simulink model "ident"  (R2018a)
settings: Solver=FixedStepAuto  StartTime=0.0  StopTime=1000  FixedStep=1e-2  MaxStep=1e-2  RelTol=1e-3
values from neighbouring files (symbols this model uses):
  B = 1    [data.m]
  C = 5    [data.m]
  V1 = 10    [data.m]
  V2 = 20    [data.m]
settings Model: Creator=User  LastModifiedBy=User

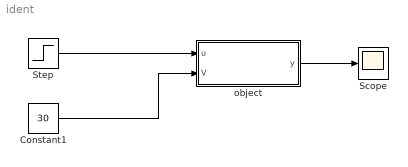
== system ident ==
  Constant1 : Constant  Value=30
  Scope : Scope
  Step : Step  SampleTime=0.01
  object : Subsystem
  wires:
  Constant1/1 -> object/2(V)
  Step/1 -> object/1(u)
  object/1(y) -> Scope/1

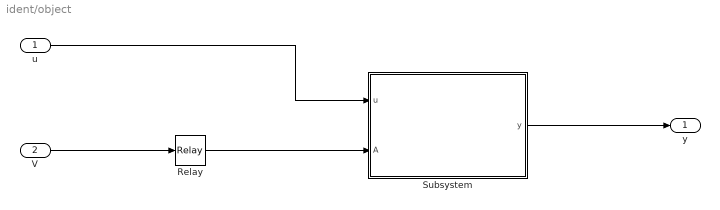
== system ident/object ==
  u : Inport
  V : Inport  Port=2
  Relay : Relay  OnSwitchValue=V2  OffSwitchValue=V1  OnOutputValue=A2  OffOutputValue=A1
  Subsystem : Subsystem
  y : Outport
  wires:
  V/1 -> Relay/1
  Relay/1 -> Subsystem/2(A)
  u/1 -> Subsystem/1(u)
  Subsystem/1(y) -> y/1

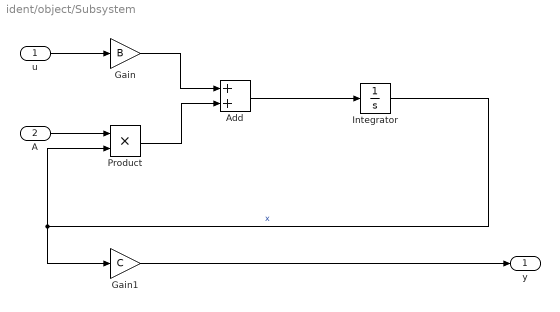
== system ident/object/Subsystem ==
  u : Inport
  A : Inport  Port=2
  Add : Sum
  Gain : Gain  Gain=B
  Gain1 : Gain  Gain=C
  Integrator : Integrator
  Product : Product
  y : Outport
  wires:
  A/1 -> Product/1
  Integrator/1 -> Gain1/1, Product/2  "x"
  u/1 -> Gain/1
  Gain/1 -> Add/1
  Product/1 -> Add/2
  Add/1 -> Integrator/1
  Gain1/1 -> y/1
